simulink model "INVCPA"  (R2022b)
settings: configuration reference "SharedConfig" (kept outside this file)
values from neighbouring files (symbols this model uses):
  PhaUACmdDialEna_C = 0.0    [INVCPA.sldd]
  PhaUACmdDialVal_C = 0.0    [INVCPA.sldd]
  PhaUBCmdDialEna_C = 0.0    [INVCPA.sldd]
  PhaUBCmdDialVal_C = 0.0    [INVCPA.sldd]
  PhaUCCmdDialEna_C = 0.0    [INVCPA.sldd]
  PhaUCCmdDialVal_C = 0.0    [INVCPA.sldd]
undefined symbols (not defined in the file or in its folder): slcm
Description:
  | Performs inverse park and clark transforms to generate phase voltage targets for dq-axis voltage targets.
settings Model: DataDictionary=INVCPA.sldd  Creator=Kevin  LastModifiedBy=Max Kolesnikov
settings ConfigSetRef: SourceName=SharedConfig

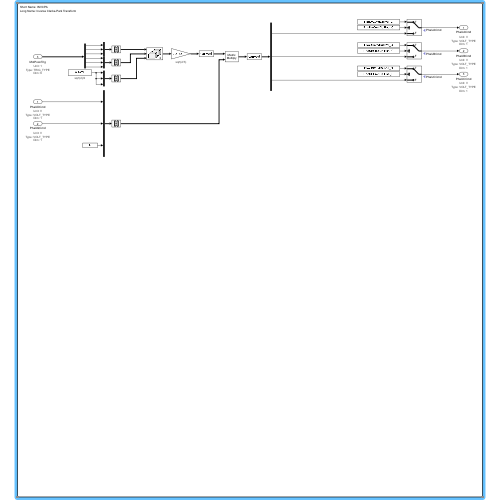
[thumbnail: Simulink's stored preview of the top-level diagram]
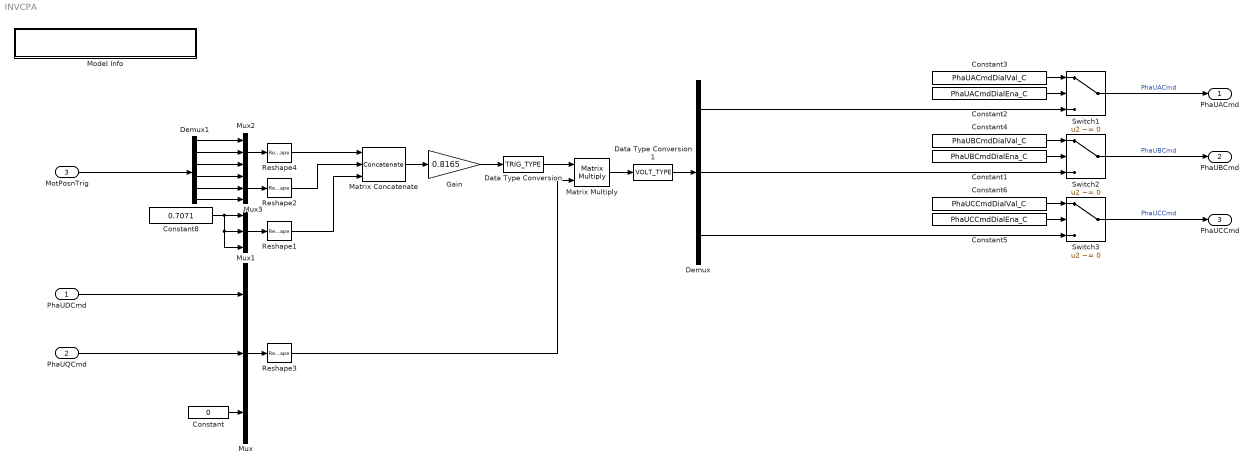
== system INVCPA ==
  PhaUDCmd : Inport  OutDataTypeStr=VOLT_TYPE  Unit=V  PortDimensions=1
      settings: AttributesFormatString=|
      | Unit: %<Unit>
      | Type: %<OutDataTypeStr>
      | Dim: %<PortDimensions>
  PhaUQCmd : Inport  Port=2  OutDataTypeStr=VOLT_TYPE  Unit=V  PortDimensions=1
      settings: AttributesFormatString=|
      | Unit: %<Unit>
      | Type: %<OutDataTypeStr>
      | Dim: %<PortDimensions>
  MotPosnTrig : Inport  Port=3  OutDataTypeStr=TRIG_TYPE  Unit=1  PortDimensions=6
      settings: AttributesFormatString=|
      | Unit: %<Unit>
      | Type: %<OutDataTypeStr>
      | Dim: %<PortDimensions>
  Constant : Constant  Value=0  OutDataTypeStr=VOLT_TYPE  LockScale=on
  Constant1 : Constant  Value=PhaUBCmdDialEna_C
  Constant2 : Constant  Value=PhaUACmdDialEna_C
  Constant3 : Constant  Value=PhaUACmdDialVal_C
  Constant4 : Constant  Value=PhaUBCmdDialVal_C
  Constant5 : Constant  Value=PhaUCCmdDialEna_C
  Constant6 : Constant  Value=PhaUCCmdDialVal_C
  Constant8 : Constant  Description=sqrt(2)/2  Value=0.7071  OutDataTypeStr=TRIG_TYPE
      settings: AttributesFormatString=%<Description>
  Data Type Conversion : DataTypeConversion  OutDataTypeStr=TRIG_TYPE  SaturateOnIntegerOverflow=off  RndMeth=Floor
  Data Type Conversion1 : DataTypeConversion  OutDataTypeStr=VOLT_TYPE  SaturateOnIntegerOverflow=off  RndMeth=Floor
  Demux : Demux  Outputs=3
  Demux1 : Demux  Outputs=6
  Gain : Gain  Description=sqrt(2/3)  Gain=0.8165
      settings: AttributesFormatString=%<Description>
  Matrix Concatenate : Concatenate  NumInputs=3  Mode=Multidimensional array  ConcatenateDimension=2
  Matrix Multiply : Product  Multiplication=Matrix(*)
  Model Info : Subsystem  LoadFcn=slcm LoadBlock;  InitFcn=slcm('UpdateAllCMBlocksInThisModelInit')  mask(CMBlock){Frame=off, DisplayStringWithTags=|, MaskDisplayString=Short Name: INVCPA\nLong Name: Inverse Clarke-Park Transform, HorizontalTextAlignment=Left, LeftAlignmentValue=0.02}
      mask DisplayStringWithTags=|
      | Short Name: %<ModelName>
      | Long Name: Inverse Clarke-Park Transform
      mask prompts: Frame "Simulink:masks:Frame_MP"; DisplayStringWithTags "Simulink:masks:DisplayStringWithTags_MP"; MaskDisplayString "Simulink:masks:MaskDisplayString_MP"; HorizontalTextAlignment "Simulink:masks:HorizontalTextAlignment_MP"; LeftAlignmentValue "Simulink:masks:LeftAlignmentValue_MP"
      mask help: Simulink:masks:CMBlock_MD
      settings: CopyFcn=slcm CopyBlock;  DeleteFcn=slcm Cancel;  PostSaveFcn=slcm('UpdateAllCMBlocksInThisModel')  NameChangeFcn=slcm Rename;  OpenFcn=slcm
      mask Display: text(slResolve(LeftAlignmentValue, gcbh), 0.5, MaskDisplayString, 'HorizontalAlignment', HorizontalTextAlignment)
  Mux{,1..3} (4 alike) : Mux  Inputs=3
  Reshape{1..4} (4 alike) : Reshape  OutputDimensionality=Column vector (2-D)
  Switch1 : Switch  Criteria=u2 ~= 0  SaturateOnIntegerOverflow=off  InputSameDT=off
  Switch2 : Switch  Criteria=u2 ~= 0  SaturateOnIntegerOverflow=off  InputSameDT=off
  Switch3 : Switch  Criteria=u2 ~= 0  SaturateOnIntegerOverflow=off  InputSameDT=off
  PhaUACmd : Outport  OutDataTypeStr=VOLT_TYPE  Unit=V  PortDimensions=1
      settings: AttributesFormatString=|
      | Unit: %<Unit>
      | Type: %<OutDataTypeStr>
      | Dim: %<PortDimensions>
  PhaUBCmd : Outport  Port=2  OutDataTypeStr=VOLT_TYPE  Unit=V  PortDimensions=1
      settings: AttributesFormatString=|
      | Unit: %<Unit>
      | Type: %<OutDataTypeStr>
      | Dim: %<PortDimensions>
  PhaUCCmd : Outport  Port=3  OutDataTypeStr=VOLT_TYPE  Unit=V  PortDimensions=1
      settings: AttributesFormatString=|
      | Unit: %<Unit>
      | Type: %<OutDataTypeStr>
      | Dim: %<PortDimensions>
  wires:
  Constant2/1 -> Switch1/2
  Switch1/1 -> PhaUACmd/1  "PhaUACmd"
  Constant3/1 -> Switch1/1
  Constant4/1 -> Switch2/1
  Switch2/1 -> PhaUBCmd/1  "PhaUBCmd"
  Constant1/1 -> Switch2/2
  Constant5/1 -> Switch3/2
  Switch3/1 -> PhaUCCmd/1  "PhaUCCmd"
  Constant6/1 -> Switch3/1
  Constant/1 -> Mux/3
  Constant8/1 -> Mux1/3, Mux1/2, Mux1/1
  Demux1/6 -> Mux3/3
  Demux1/5 -> Mux3/2
  Demux1/3 -> Mux2/3
  Demux1/2 -> Mux2/2
  Mux2/1 -> Reshape4/1
  Demux1/4 -> Mux3/1
  Demux/2 -> Switch2/3
  Demux/3 -> Switch3/3
  Demux/1 -> Switch1/3
  Demux1/1 -> Mux2/1
  Gain/1 -> Data Type Conversion/1
  Matrix Concatenate/1 -> Gain/1
  Mux/1 -> Reshape3/1
  MotPosnTrig/1 -> Demux1/1
  Mux1/1 -> Reshape1/1
  Mux3/1 -> Reshape2/1
  Reshape3/1 -> Matrix Multiply/2
  Reshape1/1 -> Matrix Concatenate/3
  Reshape2/1 -> Matrix Concatenate/2
  Reshape4/1 -> Matrix Concatenate/1
  Matrix Multiply/1 -> Data Type Conversion1/1
  Data Type Conversion/1 -> Matrix Multiply/1
  Data Type Conversion1/1 -> Demux/1
  PhaUQCmd/1 -> Mux/2
  PhaUDCmd/1 -> Mux/1

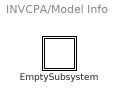
== system INVCPA/Model Info ==
  EmptySubsystem : Subsystem

== system INVCPA/Model Info/EmptySubsystem ==
